simulink model "s0511_rollsensorfusion_CF_withBank"  (R2021a)
settings: Solver=FixedStepAuto  StartTime=0.0  StopTime=10.0  RelTol=1e-3  EnableMultiTasking=on
undefined symbols (not defined in the file or in its folder): Ts
libraries: CarMaker4SL x16, dspfdesign x1
settings Model: Creator=jason  LastModifiedBy=jason
settings ModelReferenceCC: ModelReferenceNumInstancesAllowed=Single

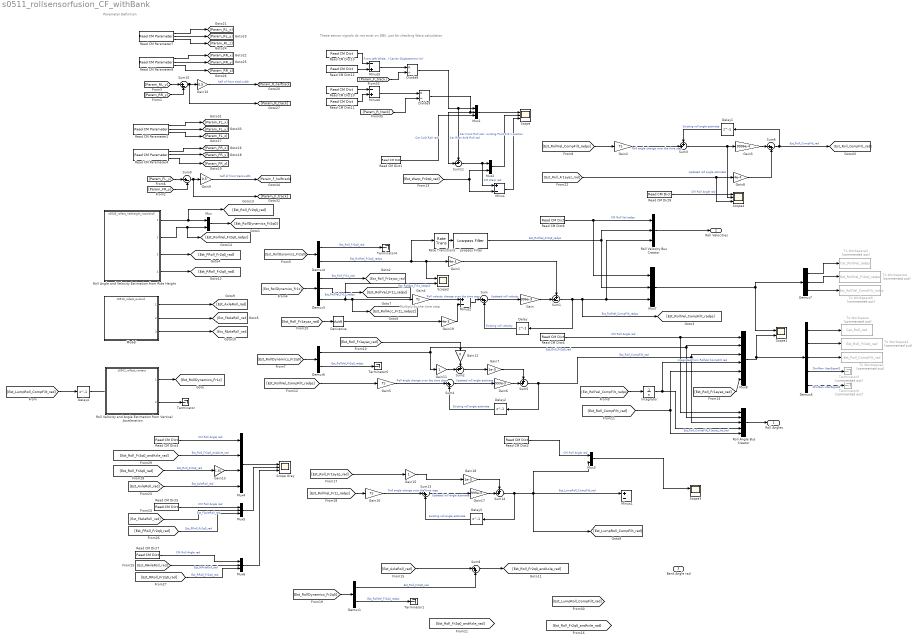
== system s0511_rollsensorfusion_CF_withBank ==
  note: These sensor signals do not exist on DBX, just for checking Warp calculation
  note: Multiply by the time step
  note: Parameter Definition
  Delay{,1..4} (5 alike) : Delay  DelayLength=1
  Demux1 : Demux  Outputs=2
      settings: DisplayOption=none
  Demux3 : Demux  Outputs=3
      settings: DisplayOption=none
  Demux4 : Demux  Outputs=2
      settings: DisplayOption=none
  Demux5 : Demux  Outputs=5
      settings: DisplayOption=none
  Demux6 : Demux  Outputs=2
      settings: DisplayOption=none
  Demux7 : Demux  Outputs=3
  Derivative : Derivative
  Divide8 : Product  Inputs=*/
  Divide9 : Product  Inputs=*/
  Gain : Gain  Gain=996e-3
  Gain1 : Gain  Gain=4e-3
  Gain10 : Gain  Gain=0.5
  Gain11 : Gain
  Gain12 : Gain  Gain=0
  Gain13 : Gain  Gain=1.35
  Gain15 : Gain
  Gain{2,4..5,16} (4 alike) : Gain  Gain=Ts
  Gain17 : Gain  Gain=999e-3
  Gain18 : Gain  Gain=1e-3
  Gain19 : Gain  Gain=4e-3
  Gain3 : Gain  Gain=9996e-4
  Gain6 : Gain  Gain=999e-3
  Gain7 : Gain  Gain=1e-3
  Gain8 : Gain  Gain=4e-4
  Gain9 : Gain  Gain=0.5
  Integrator : Integrator
  Lowpass Filter : dspfdesign/Lowpass Filter  FilterType=FIR  DesignForMinimumOrder=on  FilterOrder=50  PassbandFrequency=1  StopbandFrequency=2000  PassbandRipple=0.1  StopbandAttenuation=180  InheritSampleRate=off  SampleRate=44100  SimulateUsing=Interpreted execution  roundingMode=Floor  coeffsDataTypeStr=fixdt(1,16)
  Minus : Sum  Inputs=+-
  Minus1 : Sum  Inputs=+-
  Minus2 : Sum  Inputs=+-
  Minus5 : Sum  Inputs=-+
  Minus6 : Sum  Inputs=-+
  Model : ModelReference  ModelNameDialog=s0510_rollest_axleroll.slx  SimulationMode=Normal  ModelReferenceVersion=1.22
  Mux : Mux  Inputs=2
  Mux{1,3,5..7} (5 alike) : Mux  Inputs=3
  Mux2 : Mux  Inputs=2
  Mux4 : Mux
  Mux8 : Mux  Inputs=6
  Rate Transition5 : RateTransition
  Read CM Dict{1..5,7..8} (7 alike) : CarMaker4SL/Read CM Dict  xname=Car.Roll  xsync=off  xstime=Continuous
  Read CM Dict10 : CarMaker4SL/Read CM Dict  xname=Car.CRL.q0  xsync=off  xstime=Continuous
  Read CM Dict11 : CarMaker4SL/Read CM Dict  xname=Car.CRR.q0  xsync=off  xstime=Continuous
  Read CM Dict12 : CarMaker4SL/Read CM Dict  xname=Car.CFR.q0  xsync=off  xstime=Continuous
  Read CM Dict13 : CarMaker4SL/Read CM Dict  xname=Car.CFL.q0  xsync=off  xstime=Continuous
  Read CM Dict6 : CarMaker4SL/Read CM Dict  xname=Car.RollVel  xsync=off  xstime=Continuous
  Read CM Parameter2 : CarMaker4SL/Read CM Parameter  xfile=Vehicle  xkey=WheelCarrier.fl.pos  xnout=3  xdefaults=eps  xmuxed=off  xstime=Continuous
      settings: SourceProductName=CarMaker4SL
  Read CM Parameter4 : CarMaker4SL/Read CM Parameter  xfile=Vehicle  xkey=WheelCarrier.fr.pos  xnout=3  xdefaults=eps  xmuxed=off  xstime=Continuous
      settings: SourceProductName=CarMaker4SL
  Read CM Parameter7 : CarMaker4SL/Read CM Parameter  xfile=Vehicle  xkey=WheelCarrier.rl.pos  xnout=3  xdefaults=eps  xmuxed=off  xstime=Continuous
      settings: SourceProductName=CarMaker4SL
  Read CM Parameter8 : CarMaker4SL/Read CM Parameter  xfile=Vehicle  xkey=WheelCarrier.rr.pos  xnout=3  xdefaults=eps  xmuxed=off  xstime=Continuous
      settings: SourceProductName=CarMaker4SL
  Roll Angle Bus Creator : BusCreator  Inputs=5  OutDataTypeStr=Bus: Est_Roll_CF
  Roll Angle and Velocity Estimation from Ride Height : ModelReference  ModelNameDialog=s0509_rollest_rideheight_noaxleroll.slx  SimulationMode=Normal  ModelReferenceVersion=1.25
  Roll Velocity Bus Creator : BusCreator  Inputs=3  OutDataTypeStr=Bus: Est_RollVel_CF
  Roll Velocity and Angle Estimation from Vertical Acceleration : ModelReference  ModelNameDialog=s0502_rollest_vertacc.slx  SimulationMode=Normal  ModelReferenceVersion=1.25
  Scope : Scope  NumInputPorts=3
  Scope Grey : Scope  NumInputPorts=3
  Scope1 : Scope  NumInputPorts=2
  Scope2 : Scope  NumInputPorts=2
  Scope3 : Scope  NumInputPorts=2
  Scope4 : Scope  NumInputPorts=3
  Sum{,4,6,8,13} (5 alike) : Sum  Inputs=|++
  Sum1 : Sum  Inputs=++-
  Sum10 : Sum  Inputs=|+-
  Sum11 : Sum  Inputs=+-|
  Sum{2..3,5,14} (4 alike) : Sum  Inputs=++|
  Sum9 : Sum  Inputs=|+-
  Terminator{,1,4..5} (4 alike) : Terminator
  Terminator3 : Terminator  Commented=on
  Terminator6 : Terminator  Commented=on
  To Workspace : ToWorkspace  Commented=on  VariableName=Car_Roll_rad  SampleTime=-1
  To Workspace1 : ToWorkspace  Commented=on  VariableName=Est_Roll_Fr2q0_rad  SampleTime=-1
  To Workspace2 : ToWorkspace  Commented=on  VariableName=Est_Roll_CompFilt_rad  SampleTime=-1
  To Workspace3 : ToWorkspace  Commented=on  VariableName=Car_RollVel_radps  SampleTime=-1
  To Workspace4 : ToWorkspace  Commented=on  VariableName=Est_RollVel_Fr2q0_radps  SampleTime=-1
  To Workspace5 : ToWorkspace  Commented=on  VariableName=Est_RollVel_CompFilt_radps  SampleTime=-1
  Roll Angles : Outport  OutDataTypeStr=Bus: Est_Roll_CF
  Roll Velocities : Outport  Port=2  OutDataTypeStr=Bus: Est_RollVel_CF
  Bank Angle rad : Outport  Port=3
  wires:
  Roll Angle and Velocity Estimation from Ride Height/2 -> [Est_RollVel_Fr2q0_radps], Mux/2
  Roll Velocity and Angle Estimation from Vertical Acceleration/1 -> [Est_RollDynamics_Fr1z]
  Roll Angle and Velocity Estimation from Ride Height/1 -> [Est_Roll_Fr2q0_rad], Mux/1
  Roll Velocity and Angle Estimation from Vertical Acceleration/2 -> Terminator/1
  Roll Angle and Velocity Estimation from Ride Height/3 -> [Est_FRoll_Fr2q0_rad]
  Mux/1 -> [Est_RollDynamics_Fr2q0]
  [Est_RollDynamics_Fr2q0] -> Demux4/1
  [Est_RollDynamics_Fr1z] -> Demux3/1
  Sum/1 -> Gain/1  "Updated roll velocity"
  Delay/1 -> Sum/2  "Existing roll velocity"
  Gain/1 -> Sum1/2
  Gain1/1 -> Sum1/1
  Demux4/2 -> Rate Transition5/1, Scope2/1, Gain1/1  "Est_RollVel_Fr2q0_radps"
  Demux3/3 -> [Est_RollAcc_Fr1z_radps2], Gain4/1, Scope2/2  "Est_RollAcc_Fr1z_radps2"
  Read CM Dict6/1 -> Mux7/1, Roll Velocity Bus Creator/1  "CM Roll Vel radps"
  Mux7/1 -> Demux7/1, Scope1/1
  Gain4/1 -> Minus2/1  "Roll velocity change over the time step"
  Lowpass Filter/1 -> Mux7/2, Roll Velocity Bus Creator/2  "Est_RollVel_Fr2q0_radps"
  Rate Transition5/1 -> Lowpass Filter/1
  Demux3/1 -> [Est_Roll_Fr1ayaz_rad]  "Est_Roll_Fr1z_rad"
  Gain5/1 -> Sum4/1  "Roll angle change over the time step"
  Sum5/1 -> Roll Angle Bus Creator/3, Mux8/3, Delay2/1  "Est_Roll_CompFilt_rad"
  Delay2/1 -> Sum4/2  "Existing roll angle estimate"
  Gain6/1 -> Sum5/2
  Sum4/1 -> Gain6/1  "Updated roll angle estimate"
  [Est_RollDynamics_Fr2q0] -> Demux6/1
  Demux6/1 -> Gain11/1, Mux8/2, Roll Angle Bus Creator/2  "Est_Roll_Fr2q0_rad"
  Gain7/1 -> Sum5/1
  Demux4/1 -> Terminator4/1  "Est_Roll_Fr2q0_rad"
  Demux6/2 -> Terminator5/1  "Est_RollVel_Fr2q0_radps"
  Read CM Dict4/1 -> Mux8/1, Roll Angle Bus Creator/1  "CM Roll Angle rad"
  [Est_RollVel_CompFilt_radps] -> Gain5/1
  Sum3/1 -> Scope4/2, Gain3/1  "Updated roll angle estimate"
  Gain2/1 -> Sum3/2  "Roll angle change over the time step"
  Delay1/1 -> Sum3/1  "Existing roll angle estimate"
  Sum6/1 -> Delay1/1, [Est_Roll_CompFilt_rad]  "Est_Roll_CompFilt_rad"
  [Est_Roll_Fr1ayaz_rad] -> Scope4/3, Gain8/1
  Gain8/1 -> Sum6/2
  Gain3/1 -> Sum6/1
  [Est_RollVel_CompFilt_radps] -> Gain2/1
  Read CM Dict8/1 -> Scope4/1  "CM Roll Angle rad"
  [Est_RollVel_CompFilt_radps] -> Integrator/1
  Integrator/1 -> Mux8/4, Roll Angle Bus Creator/4  "Integrated from RollVel CompFilt rad"
  [Est_Roll_CompFilt_rad] -> Roll Angle Bus Creator/5, Mux8/5  "Est_Roll_CompFilt_F1ayaz_Int_rad"
  [Est_Roll_Fr1ayaz_rad] -> Gain12/1
  Gain11/1 -> Sum2/2
  Gain12/1 -> Sum2/1
  Sum2/1 -> Gain7/1
  Demux5/1 -> To Workspace/1
  Demux5/2 -> To Workspace1/1
  Demux5/3 -> To Workspace2/1
  Demux5/4 -> Terminator3/1  "DrivMan UserSignal1"
  Demux5/5 -> Terminator6/1  "DrivMan UserSignal2"
  Demux7/1 -> To Workspace3/1
  Demux7/2 -> To Workspace4/1
  Demux7/3 -> To Workspace5/1
  Sum1/1 -> Delay/1, Roll Velocity Bus Creator/3, Mux7/3, [Est_RollVel_CompFilt_radps]  "Est_RollVel_CompFilt_radps"
  Roll Velocity Bus Creator/1 -> Roll Velocities/1
  Roll Angle Bus Creator/1 -> Roll Angles/1
  Mux8/1 -> Demux5/1, Scope1/2
  Demux3/2 -> [Est_RollVel_Fr1z_radps]  "Est_RollVel_Fr1z_radps"
  Read CM Parameter2/3 -> [Param_FL_z]
  Gain9/1 -> [Param_F_halftrack]  "half of front trackwidth"
  Read CM Parameter2/2 -> [Param_FL_y]
  Read CM Parameter2/1 -> [Param_FL_x]
  Read CM Parameter8/1 -> [Param_RR_x]
  [Param_FR_y] -> Sum9/2
  Read CM Parameter4/1 -> [Param_FR_x]
  Read CM Parameter7/2 -> [Param_RL_y]
  Read CM Parameter7/3 -> [Param_RL_z]
  [Param_RL_y] -> Sum10/1
  Read CM Parameter8/3 -> [Param_RR_z]
  Read CM Parameter7/1 -> [Param_RL_x]
  Read CM Parameter8/2 -> [Param_RR_y]
  Read CM Parameter4/3 -> [Param_FR_z]
  Gain10/1 -> [Param_R_halftrack]  "half of front trackwidth"
  [Param_RR_y] -> Sum10/2
  [Param_FL_y] -> Sum9/1
  Sum10/1 -> Gain10/1, [Param_R_track]
  Sum9/1 -> Gain9/1, [Param_F_track]
  Read CM Parameter4/2 -> [Param_FR_y]
  Divide8/1 -> Mux1/1, Sum11/1  "Car Front Roll rad, from Mounting Point Fr0 z position"
  Divide9/1 -> Sum11/2, Mux1/2  "Car Rear Axle Roll rad"
  Read CM Dict1/1 -> Mux1/3  "Car CoG Roll rad"
  Mux1/1 -> Scope/1
  [Est_Warp_Fr2q0_rad] -> Minus/2, Mux2/2
  Sum11/1 -> Mux2/1, Minus/1  "CM Warp rad"
  Mux2/1 -> Scope/2
  Minus/1 -> Scope/3
  Minus6/1 -> Divide9/1
  [Param_F_track] -> Divide8/2
  Read CM Dict10/1 -> Minus6/1
  Read CM Dict13/1 -> Minus5/1  "Front Left Wheel Carrier Displacement (m)"
  Read CM Dict11/1 -> Minus6/2
  [Param_R_track] -> Divide9/2
  Minus5/1 -> Divide8/1
  Read CM Dict12/1 -> Minus5/2
  [Est_Roll_Fr1ayaz_rad] -> Mux8/6
  [Est_Roll_Fr1ayaz_rad] -> Gain15/1
  Gain16/1 -> Sum13/1  "Roll angle change over the time step"
  Delay3/1 -> Sum13/2  "Existing roll angle estimate"
  Gain18/1 -> Sum14/1
  Gain17/1 -> Sum14/2
  Gain15/1 -> Gain18/1
  Sum14/1 -> Minus1/1, Mux3/3, [Est_LumpRoll_CompFilt_rad], Delay3/1  "Est_LumpRoll_CompFilt_rad"
  Sum13/1 -> Gain17/1  "Updated roll angle estimate"
  Read CM Dict2/1 -> Mux3/1  "CM Roll Angle rad"
  Mux3/1 -> Scope3/1
  [Est_RollVel_Fr1z_radps] -> Gain16/1
  [Est_Roll_Fr1ayaz_rad] -> Derivative/1
  Derivative/1 -> Gain19/1
  Gain19/1 -> Minus2/2
  Minus2/1 -> Sum/1
  Delay4/1 -> ?
  [Est_LumpRoll_CompFilt_rad] -> Delay4/1
  Demux1/1 -> Sum8/2  "Est_Roll_Fr2q0_rad"
  Demux1/2 -> Terminator1/1  "Est_RollVel_Fr2q0_radps"
  [Est_RollDynamics_Fr2q0] -> Demux1/1
  Model/2 -> [Est_FAxleRoll_rad]
  Model/1 -> [Est_AxleRoll_rad]
  Model/3 -> [Est_RAxleRoll_rad]
  [Est_AxleRoll_rad] -> Sum8/1
  Sum8/1 -> [Est_Roll_Fr2q0_andAxle_rad]
  Roll Angle and Velocity Estimation from Ride Height/4 -> [Est_RRoll_Fr2q0_rad]
  Read CM Dict3/1 -> Mux4/1  "CM Roll Angle rad"
  [Est_Roll_Fr2q0_andAxle_rad] -> Mux4/2  "Est_Roll_Fr2q0_andAxle_rad"
  [Est_Roll_Fr2q0_rad] -> Gain13/1  "Est_Roll_Fr2q0_rad"
  [Est_AxleRoll_rad] -> Mux4/4  "Est_AxleRoll_rad"
  Mux4/1 -> Scope Grey/1
  [Est_FAxleRoll_rad] -> Mux5/2  "Est_FAxleRoll_rad"
  [Est_FRoll_Fr2q0_rad] -> Mux5/3  "Est_FRoll_Fr2q0_rad"
  Read CM Dict5/1 -> Mux5/1  "CM Roll Angle rad"
  Read CM Dict7/1 -> Mux6/1  "CM Roll Angle rad"
  [Est_RAxleRoll_rad] -> Mux6/2  "Est_RAxleRoll_rad"
  [Est_RRoll_Fr2q0_rad] -> Mux6/3  "Est_RRoll_Fr2q0_rad"
  Mux5/1 -> Scope Grey/2
  Mux6/1 -> Scope Grey/3
  Gain13/1 -> Mux4/3
